simulink model "Experiment_AERO_pitch_channel"  (Simulink 9.1)
settings: Solver=ode4  StartTime=0.0  StopTime=35  FixedStep=0.001  RelTol=1e-3  EnableMultiTasking=on
InitFcn:
  | Parameters_and_initial_conditions
values from neighbouring files (symbols this model uses):
  a1 = -Ksp/Jp    (= -3.27334590734)    [Parameters_and_initial_conditions.m]
  a2 = -Dp/Jp    (= -0.354944459971)    [Parameters_and_initial_conditions.m]
  Dp = 0.007768621416960    (= 0.00776862141696)    [Parameters_and_initial_conditions.m]
  Dp_static = Dp*0.05    (= 0.000388431070848)    [Parameters_and_initial_conditions.m]
  Dy = 0.0220    (= 0.022)    [Parameters_and_initial_conditions.m]
  Jp = J_body + 2*J_prop    (= 0.0218868648283)    [Parameters_and_initial_conditions.m]
  Jy = J_body + 2*J_prop + J_yoke    (= 0.0219920648283)    [Parameters_and_initial_conditions.m]
  kd = 3    [Parameters_and_initial_conditions.m]
  kp = 5    [Parameters_and_initial_conditions.m]
  Kpp = 9.971955650940002e-04    (= 0.000997195565094)    [Parameters_and_initial_conditions.m]
  Kpy = 0.0021    [Parameters_and_initial_conditions.m]
  Ksp = 0.071643279410402    (= 0.0716432794104)    [Parameters_and_initial_conditions.m]
  Kyp = -0.0027    [Parameters_and_initial_conditions.m]
  Kyy = 0.0022    [Parameters_and_initial_conditions.m]
  PitchAxisEnable = 1    [Parameters_and_initial_conditions.m]
  PitchMotorEnable = 1    [Parameters_and_initial_conditions.m]
  psi_dot_initial = 0.0    (= 0)    [Parameters_and_initial_conditions.m]
  psi_initial = 0.0    (= 0)    [Parameters_and_initial_conditions.m]
  T_1 = 1/2*eps^2    (= 0.00125)    [Parameters_and_initial_conditions.m]
  T_2 = 3/2*eps    (= 0.075)    [Parameters_and_initial_conditions.m]
  T_passive = 0.5    [Parameters_and_initial_conditions.m]
  theta_dot_initial = 0.0    (= 0)    [Parameters_and_initial_conditions.m]
  theta_initial = 0.0    (= 0)    [Parameters_and_initial_conditions.m]
  YawAxisEnable = 0    [Parameters_and_initial_conditions.m]
  YawMotorEnable = 0    [Parameters_and_initial_conditions.m]
libraries: quarc_library x7, simulink_extras x5, quanser_aero x1
settings Model: Creator=MLevis  LastModifiedBy=DELL  SimulationMode=external  ExtModeTrigDuration=5000
settings SolverCC: PositivePriorityOrder=on
settings DataIOCC: LimitDataPoints=on
settings DebuggingCC: UnderspecifiedInitializationDetection=Simplified  MergeDetectMultiDrivingBlocksExec=error  SolverPrmCheckMsg=warning
settings RTWCC: SystemTargetFile=quarc_win64.tlc  TemplateMakefile=quarc_default_tmf  Description=QUARC Win64 Target
settings STFCustomTargetCC: TargetPreCompLibLocation=C:\PROGRA~3\QUARC\lib\2018a\win64\release  ConcurrentExecutionCompliant=on  GeneratePreprocessorConditionals=Disable all  SystemTargetFile=quarc_win64.tlc
settings GRTTargetCC: TargetPreCompLibLocation=C:\PROGRA~3\QUARC\lib\2018a\win64\release  ParMdlRefBuildCompliant=off  CompOptLevelCompliant=off  GeneratePreprocessorConditionals=Disable all  MatFileLogging=off  CPPClassGenCompliant=off  UseToolchainInfoCompliant=off  ExtMode=on  ExtModeMexFile=quarc_comm
settings ConfigComp: CovSFcnEnable=off

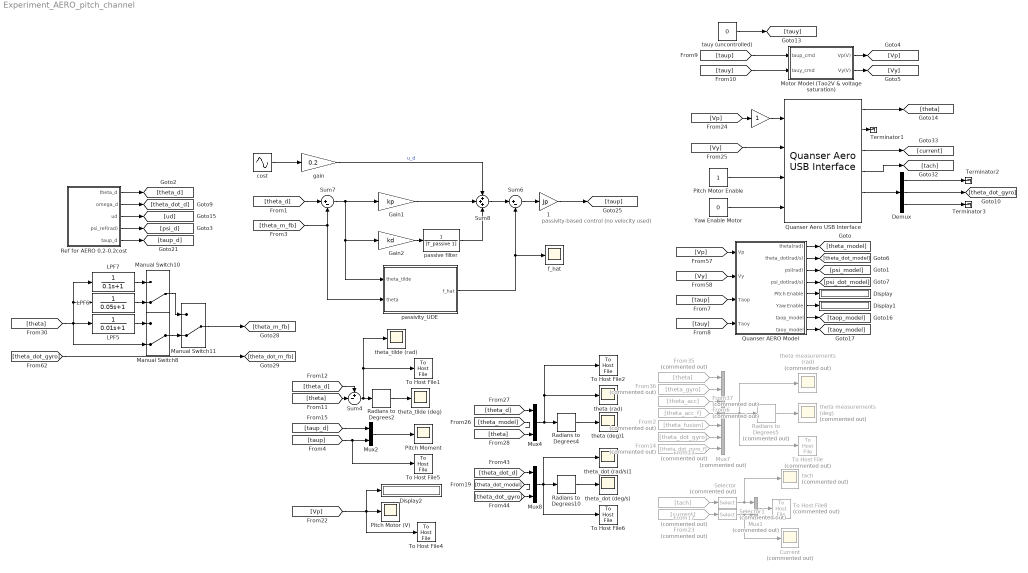
== system Experiment_AERO_pitch_channel ==
  note: passivity-based control (no velocity used)
  " " : Gain
  " 1" : Gain  Gain=Jp
  Current : Scope  Commented=on
  Demux : Demux  Outputs=3
  Display : Display
  Display1 : Display
  Display2 : Display
  From13 : From  Commented=on  GotoTag=theta_dot_gyro
  From14 : From  Commented=on  GotoTag=theta_dot_gyro_f
  From17 : From  Commented=on  GotoTag=tach
  From2 : From  Commented=on  GotoTag=theta_fusion
  From23 : From  Commented=on  GotoTag=current
  From35 : From  Commented=on  GotoTag=theta
  From36 : From  Commented=on  GotoTag=theta_gyro
  From37 : From  Commented=on  GotoTag=theta_acc
  From6 : From  Commented=on  GotoTag=theta_acc_f
  Gain1 : Gain  Gain=kp
  Gain2 : Gain  Gain=kd
  LPF5 : TransferFcn  Denominator=[0.01 1]
  LPF6 : TransferFcn  Denominator=[0.05 1]
  LPF7 : TransferFcn  Denominator=[0.1 1]
  Manual Switch10 : ManualSwitch  CurrentSetting=0
  Manual Switch11 : ManualSwitch  CurrentSetting=0
  Manual Switch8 : ManualSwitch  CurrentSetting=0
  Motor Model (Tao2V & voltage saturation) : Subsystem
  Mux1 : Mux  Commented=on  Inputs=2
  Mux2 : Mux  Inputs=2
  Mux4 : Mux  Inputs=3
  Mux7 : Mux  Commented=on  Inputs=7
  Mux8 : Mux  Inputs=3
  Pitch Moment : Scope
  Pitch Motor (V) : Scope
  Pitch Motor Enable : Constant
  Quanser AERO Model : Subsystem
  Quanser Aero USB Interface : quanser_aero/Quanser Aero USB Interface
  Radians to Degrees10 : simulink_extras/Transformations/Radians to Degrees
  Radians to Degrees2 : simulink_extras/Transformations/Radians to Degrees
  Radians to Degrees4 : simulink_extras/Transformations/Radians to Degrees
  Radians to Degrees5 : simulink_extras/Transformations/Radians to Degrees  Commented=on
  Ref for AERO 0.2-0.2cost : Subsystem
  Selector : Selector  Commented=on  InputPortWidth=2  IndexOptions=Index vector (dialog)  Indices=[1]  OutputSizes=1
  Selector1 : Selector  Commented=on  InputPortWidth=2  IndexOptions=Index vector (dialog)  Indices=[1]  OutputSizes=1
  Sum4 : Sum  Inputs=+-|
  Sum6 : Sum  Inputs=|+-
  Sum7 : Sum  Inputs=|+-
  Sum8 : Sum  Inputs=+++
  Terminator1 : Terminator
  Terminator2 : Terminator
  Terminator3 : Terminator
  To Host File : quarc_library/Sinks/To Host/To Host File  Commented=on  file_name=Log_Sensor_Measurements.mat  variable_name=Log_Sensor_Measurements  decimation=1  sample_time=-1  file_format=MAT-file v.5  options=No header or footer  append=off  final_file_name=Log_Sensor_Measurements.mat  bitrate=2000000
  To Host File1 : quarc_library/Sinks/To Host/To Host File  file_name=Log_Tracking_Err.mat  variable_name=Log_Tracking_Err  decimation=1  sample_time=-1  file_format=MAT-file v.5  options=No header or footer  append=off  final_file_name=Log_Tracking_Err.mat  bitrate=2000000
  To Host File2 : quarc_library/Sinks/To Host/To Host File  file_name=Log_Theta_Response.mat  variable_name=Log_Theta_Response  decimation=1  sample_time=-1  file_format=MAT-file v.5  options=No header or footer  append=off  final_file_name=Log_Theta_Response.mat  bitrate=2000000
  To Host File4 : quarc_library/Sinks/To Host/To Host File  file_name=Log_Input_Voltage.mat  variable_name=Log_Input_Voltage  decimation=1  sample_time=-1  file_format=MAT-file v.5  options=No header or footer  append=off  final_file_name=Log_Input_Voltage.mat  bitrate=2000000
  To Host File5 : quarc_library/Sinks/To Host/To Host File  file_name=Log_Input_Torque.mat  variable_name=Log_Input_Torque  decimation=1  sample_time=-1  file_format=MAT-file v.5  options=No header or footer  append=off  final_file_name=Log_Input_Torque.mat  bitrate=2000000
  To Host File6 : quarc_library/Sinks/To Host/To Host File  file_name=Log_Theta_dot_Response.mat  variable_name=Log_Theta_dot_Response  decimation=1  sample_time=-1  file_format=MAT-file v.5  options=No header or footer  append=off  final_file_name=Log_Theta_dot_Response.mat  bitrate=2000000
  To Host File8 : quarc_library/Sinks/To Host/To Host File  Commented=on  file_name=Log_Tach_Current.mat  variable_name=Log_Tach_Current  decimation=1  sample_time=-1  file_format=MAT-file v.5  options=No header or footer  append=off  final_file_name=Log_Tach_Current.mat  bitrate=2000000
  Yaw Enable Motor : Constant  Value=0
  cost : Sin  Phase=pi/2  SampleTime=0
  f_hat : Scope
  gain : Gain  Gain=0.2
  passive filter : TransferFcn  Denominator=[T_passive 1]
  passivity_UDE : Subsystem
  tach : Scope  Commented=on
  tauy (uncontrolled) : Constant  Value=0
  theta (deg)1 : Scope
  theta (rad) : Scope
  theta measurements (deg) : Scope  Commented=on
  theta measurements (rad) : Scope  Commented=on
  theta_dot (deg/s) : Scope
  theta_dot (rad/s)1 : Scope
  theta_tilde (deg) : Scope
  theta_tilde (rad) : Scope
  wires:
  Quanser AERO Model/3(psi(rad)) -> [psi_model]
  Quanser AERO Model/1(theta(rad)) -> [theta_model]
  Mux2/1 -> Pitch Moment/1
  Quanser AERO Model/2(theta_dot(rad/s)) -> [theta_dot_model]
  Quanser AERO Model/4(psi_dot(rad/s)) -> [psi_dot_model]
  Quanser AERO Model/5(Pitch Enable) -> Display/1
  Quanser AERO Model/6(Yaw Enable) -> Display1/1
  Motor Model (Tao2V & voltage saturation)/1(Vp(V)) -> [Vp]
  Motor Model (Tao2V & voltage saturation)/2(Vy(V)) -> [Vy]
  [tauy] -> Motor Model (Tao2V & voltage saturation)/2(tauy_cmd)
  [taup] -> Motor Model (Tao2V & voltage saturation)/1(taup_cmd)
  [theta_d] -> Sum4/1
  [theta] -> Sum4/2
  Sum4/1 -> To Host File1/1, theta_tilde (rad)/1, Radians to Degrees2/1
  Radians to Degrees2/1 -> theta_tilde (deg)/1
  [taup] -> To Host File5/1, Mux2/2
  [taup_d] -> Mux2/1
  tauy (uncontrolled)/1 -> [tauy]
  [Vp] -> Display2/1, To Host File4/1, Pitch Motor (V)/1
  Quanser Aero USB Interface/5 -> Demux/1
  Yaw Enable Motor/1 -> Quanser Aero USB Interface/4
  Quanser Aero USB Interface/4 -> [tach]
  Quanser Aero USB Interface/1 -> [theta]
  Demux/3 -> Terminator3/1
  Pitch Motor Enable/1 -> Quanser Aero USB Interface/3
  Quanser Aero USB Interface/3 -> [current]
  [Vy] -> Quanser Aero USB Interface/2
  Demux/1 -> Terminator2/1
  Demux/2 -> [theta_dot_gyro]
  Quanser Aero USB Interface/2 -> Terminator1/1
  " "/1 -> Quanser Aero USB Interface/1
  Radians to Degrees4/1 -> theta (deg)1/1
  [theta_model] -> ?
  [theta_d] -> Mux4/1
  [theta] -> Mux4/3
  Quanser AERO Model/7(taop_model) -> [taop_model]
  Quanser AERO Model/8(taoy_model) -> [taoy_model]
  From35/1 -> Mux7/1
  From36/1 -> Mux7/2
  From37/1 -> Mux7/3
  Radians to Degrees5/1 -> theta measurements (deg)/1
  Radians to Degrees10/1 -> theta_dot (deg/s)/1
  [theta_dot_model] -> ?
  Mux8/1 -> Radians to Degrees10/1, To Host File6/1, theta_dot (rad/s)1/1
  [theta_dot_gyro] -> Mux8/3
  [theta_dot_d] -> Mux8/1
  From6/1 -> Mux7/4
  Mux7/1 -> To Host File/1, theta measurements (rad)/1, Radians to Degrees5/1
  [taup] -> Quanser AERO Model/3(Taop)
  [tauy] -> Quanser AERO Model/4(Taoy)
  [Vp] -> Quanser AERO Model/1(Vp)
  [Vy] -> Quanser AERO Model/2(Vy)
  [theta_dot_gyro] -> [theta_dot_m_fb]
  Mux4/1 -> Radians to Degrees4/1, To Host File2/1, theta (rad)/1
  From2/1 -> Mux7/5
  From13/1 -> Mux7/6
  From14/1 -> Mux7/7
  From17/1 -> Selector/1
  Mux1/1 -> To Host File8/1
  From23/1 -> Selector1/1
  Selector/1 -> tach/1, Mux1/1
  Selector1/1 -> Current/1, Mux1/2
  Ref for AERO 0.2-0.2cost/1(theta_d) -> [theta_d]
  Ref for AERO 0.2-0.2cost/2(omega_d) -> [theta_dot_d]
  Ref for AERO 0.2-0.2cost/4(psi_ref(rad)) -> [psi_d]
  Ref for AERO 0.2-0.2cost/3(ud) -> [ud]
  Manual Switch11/1 -> [theta_m_fb]
  [theta] -> LPF5/1, Manual Switch8/2, LPF7/1, LPF6/1
  Ref for AERO 0.2-0.2cost/5(taup_d) -> [taup_d]
  LPF5/1 -> Manual Switch8/1
  LPF6/1 -> Manual Switch10/2
  LPF7/1 -> Manual Switch10/1
  Manual Switch10/1 -> Manual Switch11/1
  Manual Switch8/1 -> Manual Switch11/2
  [Vp] -> " "/1
  [theta_m_fb] -> passivity_UDE/2(theta), Sum7/2
  passivity_UDE/1(f_hat) -> f_hat/1, Sum6/2
  Gain1/1 -> Sum8/2
  [theta_d] -> Sum7/1
  Gain2/1 -> passive filter/1
  Sum8/1 -> Sum6/1
  Sum7/1 -> passivity_UDE/1(theta_tilde), Gain2/1, Gain1/1
  Sum6/1 -> " 1"/1
  passive filter/1 -> Sum8/3
  gain/1 -> Sum8/1  "u_d"
  " 1"/1 -> [taup]
  cost/1 -> gain/1

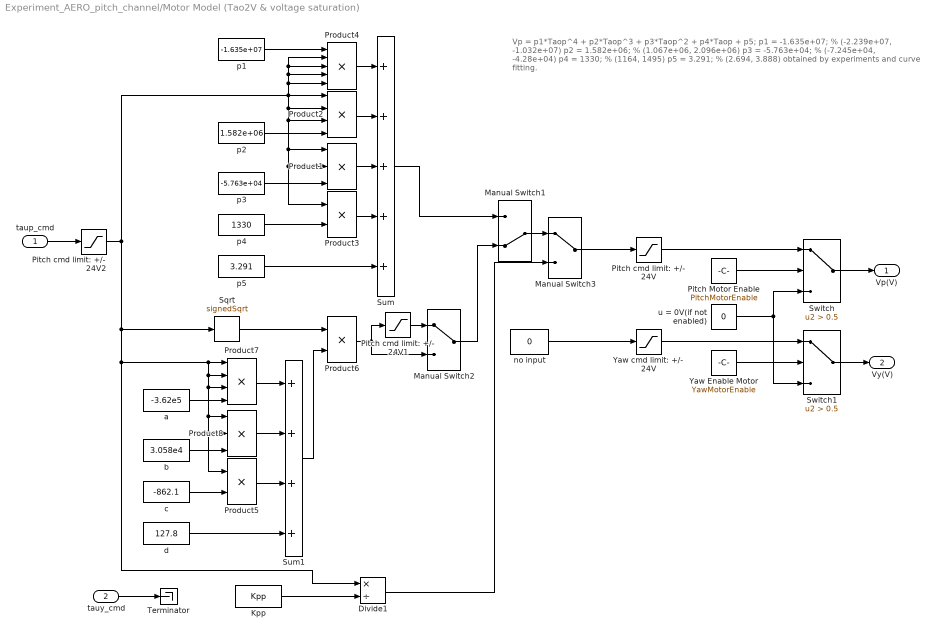
== system Experiment_AERO_pitch_channel/Motor Model (Tao2V & voltage saturation) ==
  note: Vp = p1*Taop^4 + p2*Taop^3 + p3*Taop^2 + p4*Taop + p5;
      | p1 = -1.635e+07; % (-2.239e+07, -1.032e+07)
      | p2 = 1.582e+06; % (1.067e+06, 2.096e+06)
      | p3 = -5.763e+04; % (-7.245e+04, -4.28e+04)
      | p4 = 1330; % (1164, 1495)
      | p5 = 3.291; % (2.694, 3.888)
      |
      | obtained by experiments and curve fitting.
  taup_cmd : Inport
  tauy_cmd : Inport  Port=2
  Divide1 : Product  Inputs=*/
  Kpp : Constant  Value=Kpp
  Manual Switch1 : ManualSwitch  CurrentSetting=0
  Manual Switch2 : ManualSwitch
  Manual Switch3 : ManualSwitch
  Pitch Motor Enable : Constant  Value=PitchMotorEnable
  Pitch cmd limit: +/- 24V : Saturate  UpperLimit=24  LowerLimit=-24
  Pitch cmd limit: +/- 24V1 : Saturate  UpperLimit=24  LowerLimit=0
  Pitch cmd limit: +/- 24V2 : Saturate  UpperLimit=0.05  LowerLimit=0
  Product1 : Product  Inputs=3
  Product2 : Product  Inputs=4
  Product3 : Product
  Product4 : Product  Inputs=5
  Product5 : Product
  Product6 : Product
  Product7 : Product  Inputs=4
  Product8 : Product  Inputs=3
  Sqrt : Sqrt  Operator=signedSqrt  SaturateOnIntegerOverflow=on
  Sum : Sum  Inputs=+++++
  Sum1 : Sum  Inputs=++++
  Switch : Switch  Criteria=u2 > Threshold  Threshold=0.5
  Switch1 : Switch  Criteria=u2 > Threshold  Threshold=0.5
  Terminator : Terminator
  Yaw Enable Motor : Constant  Value=YawMotorEnable
  Yaw cmd limit: +/- 24V : Saturate  UpperLimit=24  LowerLimit=-24
  a : Constant  Value=-3.62e5
  b : Constant  Value=3.058e4
  c : Constant  Value=-862.1
  d : Constant  Value=127.8
  no input : Constant  Value=0
  p1 : Constant  Value=-1.635e+07
  p2 : Constant  Value=1.582e+06
  p3 : Constant  Value=-5.763e+04
  p4 : Constant  Value=1330
  p5 : Constant  Value=3.291
  u = 0V(if not enabled) : Constant  Value=0
  Vp(V) : Outport
  Vy(V) : Outport  Port=2
  wires:
  Pitch Motor Enable/1 -> Switch/2
  Yaw Enable Motor/1 -> Switch1/2
  Switch/1 -> Vp(V)/1
  Switch1/1 -> Vy(V)/1
  Yaw cmd limit: +/- 24V/1 -> Switch1/1
  Pitch cmd limit: +/- 24V/1 -> Switch/1
  u = 0V(if not enabled)/1 -> Switch1/3, Switch/3
  tauy_cmd/1 -> Terminator/1
  p2/1 -> Product2/4
  no input/1 -> Yaw cmd limit: +/- 24V/1
  Product2/1 -> Sum/2
  p3/1 -> Product1/3
  p4/1 -> Product3/2
  Kpp/1 -> Divide1/2
  Product1/1 -> Sum/3
  Product3/1 -> Sum/4
  p5/1 -> Sum/5
  Sum/1 -> Manual Switch1/1
  Product4/1 -> Sum/1
  p1/1 -> Product4/1
  Manual Switch3/1 -> Pitch cmd limit: +/- 24V/1
  a/1 -> Product7/4
  b/1 -> Product8/3
  Sum1/1 -> Product6/2
  Sqrt/1 -> Product6/1
  Product6/1 -> Pitch cmd limit: +/- 24V1/1, Manual Switch2/2
  Manual Switch1/1 -> Manual Switch3/1
  Divide1/1 -> Manual Switch3/2
  d/1 -> Sum1/4
  Product7/1 -> Sum1/1
  Product8/1 -> Sum1/2
  Product5/1 -> Sum1/3
  c/1 -> Product5/2
  taup_cmd/1 -> Pitch cmd limit: +/- 24V2/1
  Pitch cmd limit: +/- 24V1/1 -> Manual Switch2/1
  Manual Switch2/1 -> Manual Switch1/2
  Pitch cmd limit: +/- 24V2/1 -> Sqrt/1, Divide1/1, Product7/1, Product7/2, Product7/3, Product8/1, Product8/2, Product5/1, Product4/5, Product4/4, Product4/3, Product4/2, Product2/1, Product3/1, Product1/2, Product1/1, Product2/3, Product2/2

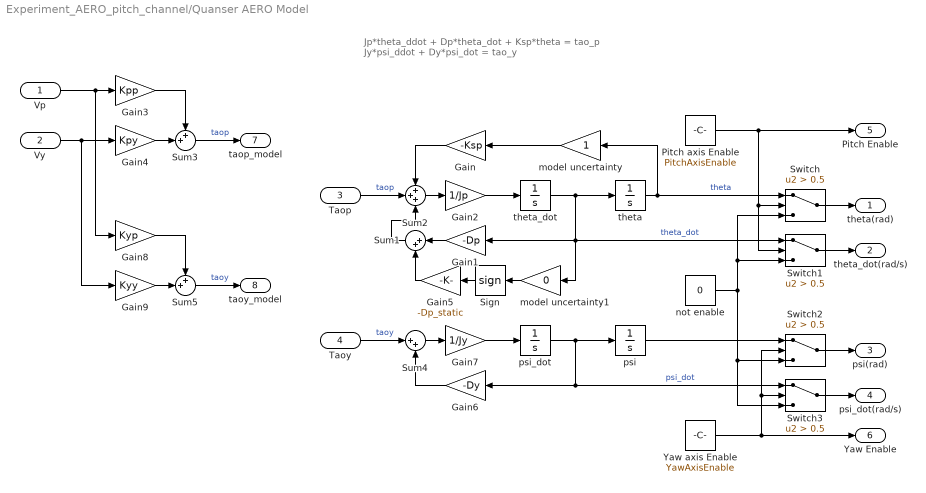
== system Experiment_AERO_pitch_channel/Quanser AERO Model ==
  note: Jp*theta_ddot + Dp*theta_dot + Ksp*theta = tao_p
      | Jy*psi_ddot + Dy*psi_dot = tao_y
  Vp : Inport
  Vy : Inport  Port=2
  Taop : Inport  Port=3
  Taoy : Inport  Port=4
  Gain : Gain  Gain=-Ksp
  Gain1 : Gain  Gain=-Dp
  Gain2 : Gain  Gain=1/Jp
  Gain3 : Gain  Gain=Kpp
  Gain4 : Gain  Gain=Kpy
  Gain5 : Gain  Gain=-Dp_static
  Gain6 : Gain  Gain=-Dy
  Gain7 : Gain  Gain=1/Jy
  Gain8 : Gain  Gain=Kyp
  Gain9 : Gain  Gain=Kyy
  Pitch axis Enable : Constant  Value=PitchAxisEnable
  Sign : Signum
  Sum1 : Sum  Inputs=|++
  Sum2 : Sum  Inputs=+++
  Sum3 : Sum  Inputs=++|
  Sum4 : Sum  Inputs=|++
  Sum5 : Sum  Inputs=++|
  Switch{,1..3} (4 alike) : Switch  Criteria=u2 > Threshold  Threshold=0.5
  Yaw axis Enable : Constant  Value=YawAxisEnable
  model uncertainty : Gain
  model uncertainty1 : Gain  Gain=0
  not enable : Constant  Value=0
  psi : Integrator  InitialCondition=psi_initial
  psi_dot : Integrator  InitialCondition=psi_dot_initial
  theta : Integrator  InitialCondition=theta_initial
  theta_dot : Integrator  InitialCondition=theta_dot_initial
  theta(rad) : Outport
  theta_dot(rad/s) : Outport  Port=2
  psi(rad) : Outport  Port=3
  psi_dot(rad/s) : Outport  Port=4
  Pitch Enable : Outport  Port=5
  Yaw Enable : Outport  Port=6
  taop_model : Outport  Port=7
  taoy_model : Outport  Port=8
  wires:
  theta_dot/1 -> model uncertainty1/1, Gain1/1, Switch1/1, theta/1  "theta_dot"
  theta/1 -> Switch/1, model uncertainty/1  "theta"
  Taop/1 -> Sum2/2  "taop"
  Gain/1 -> Sum2/1
  Gain1/1 -> Sum1/1
  Sum2/1 -> Gain2/1
  Gain2/1 -> theta_dot/1
  Gain3/1 -> Sum3/1
  Gain4/1 -> Sum3/2
  psi_dot/1 -> psi/1, Gain6/1, Switch3/1  "psi_dot"
  psi/1 -> Switch2/1
  Taoy/1 -> Sum4/1  "taoy"
  Sum4/1 -> Gain7/1
  Gain7/1 -> psi_dot/1
  Gain8/1 -> Sum5/1
  Gain9/1 -> Sum5/2
  Vp/1 -> Gain8/1, Gain3/1
  Vy/1 -> Gain9/1, Gain4/1
  Gain6/1 -> Sum4/2
  Pitch axis Enable/1 -> Pitch Enable/1, Switch1/2, Switch/2
  Switch/1 -> theta(rad)/1
  Switch1/1 -> theta_dot(rad/s)/1
  not enable/1 -> Switch1/3, Switch/3, Switch3/3, Switch2/3
  Switch2/1 -> psi(rad)/1
  Switch3/1 -> psi_dot(rad/s)/1
  Yaw axis Enable/1 -> Yaw Enable/1, Switch2/2, Switch3/2
  model uncertainty/1 -> Gain/1
  Sum1/1 -> Sum2/3
  Gain5/1 -> Sum1/2
  Sign/1 -> Gain5/1
  model uncertainty1/1 -> Sign/1
  Sum3/1 -> taop_model/1  "taop"
  Sum5/1 -> taoy_model/1  "taoy"

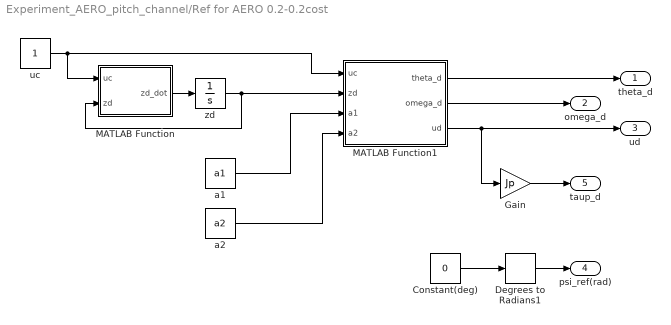
== system Experiment_AERO_pitch_channel/Ref for AERO 0.2-0.2cost ==
  Constant(deg) : Constant  Value=0
  Degrees to Radians1 : simulink_extras/Transformations/Degrees to Radians
  Gain : Gain  Gain=Jp
  MATLAB Function : MATLAB Function  TreatAsAtomicUnit=on
  MATLAB Function1 : MATLAB Function  TreatAsAtomicUnit=on
  a1 : Constant  Value=a1
  a2 : Constant  Value=a2
  uc : Constant
  zd : Integrator  InitialCondition=[0;0]
  theta_d : Outport
  omega_d : Outport  Port=2
  ud : Outport  Port=3
  psi_ref(rad) : Outport  Port=4
  taup_d : Outport  Port=5
  wires:
  MATLAB Function1/1(theta_d) -> theta_d/1
  MATLAB Function1/3(ud) -> ud/1, Gain/1
  MATLAB Function1/2(omega_d) -> omega_d/1
  a2/1 -> MATLAB Function1/4(a2)
  a1/1 -> MATLAB Function1/3(a1)
  uc/1 -> MATLAB Function/1(uc), MATLAB Function1/1(uc)
  zd/1 -> MATLAB Function/2(zd), MATLAB Function1/2(zd)
  MATLAB Function/1(zd_dot) -> zd/1
  Constant(deg)/1 -> Degrees to Radians1/1
  Degrees to Radians1/1 -> psi_ref(rad)/1
  Gain/1 -> taup_d/1

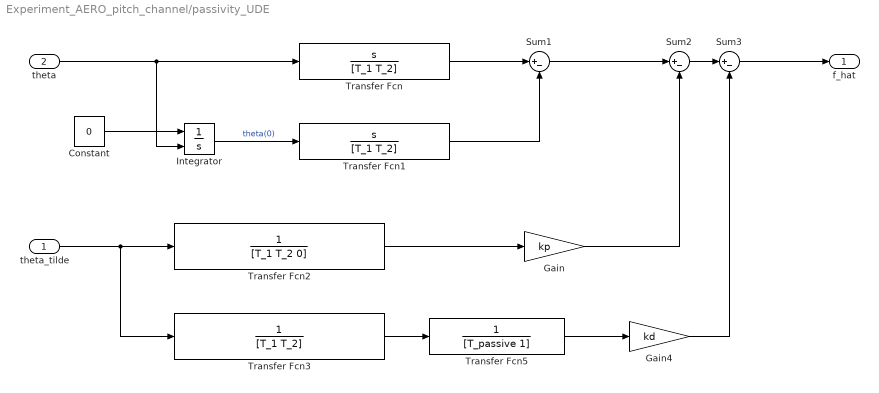
== system Experiment_AERO_pitch_channel/passivity_UDE ==
  theta_tilde : Inport
  theta : Inport  Port=2
  Constant : Constant  Value=0
  Gain : Gain  Gain=kp
  Gain4 : Gain  Gain=kd
  Integrator : Integrator  InitialConditionSource=external
  Sum1 : Sum  Inputs=|+-
  Sum2 : Sum  Inputs=|+-
  Sum3 : Sum  Inputs=|+-
  Transfer Fcn : TransferFcn  Numerator=[1 0]  Denominator=[T_1 T_2]
  Transfer Fcn1 : TransferFcn  Numerator=[1 0]  Denominator=[T_1 T_2]
  Transfer Fcn2 : TransferFcn  Denominator=[T_1 T_2 0]
  Transfer Fcn3 : TransferFcn  Denominator=[T_1 T_2]
  Transfer Fcn5 : TransferFcn  Denominator=[T_passive 1]
  f_hat : Outport
  wires:
  theta/1 -> Integrator/2, Transfer Fcn/1
  Constant/1 -> Integrator/1
  Integrator/1 -> Transfer Fcn1/1  "theta(0)"
  Transfer Fcn/1 -> Sum1/1
  Transfer Fcn1/1 -> Sum1/2
  Transfer Fcn2/1 -> Gain/1
  theta_tilde/1 -> Transfer Fcn3/1, Transfer Fcn2/1
  Sum2/1 -> Sum3/1
  Gain/1 -> Sum2/2
  Transfer Fcn3/1 -> Transfer Fcn5/1
  Transfer Fcn5/1 -> Gain4/1
  Gain4/1 -> Sum3/2
  Sum3/1 -> f_hat/1
  Sum1/1 -> Sum2/1

== matlab function Ref for AERO 0.2-0.2cost/MATLAB Function ==
  data: uc input double; zd_dot output double; zd input double
function zd_dot = ref(uc,zd)
Ad = [0 1;-1 0];
Bd = [0; 1];
zd_dot = Ad*zd + Bd*uc;

== matlab function Ref for AERO 0.2-0.2cost/MATLAB Function1 ==
  data: uc input double; zd input double; theta_d output double; omega_d output double; ud output double; a1 input double; a2 input double
function [theta_d, omega_d, ud] = fcn(uc,zd,a1,a2)
Ad = [0 1;-1 0];
Bd = [0; 1];
Cd = [0.2 0];
uc_dot = 0;
w = 0;
theta_d = Cd*zd;
omega_d = Cd*Ad*zd + Cd*Bd*uc;
ud = Cd*Ad*Ad*zd + Cd*Ad*Bd*uc + Cd*Bd*uc_dot - a1*Cd*zd - a2*Cd*Ad*zd - w;
